simulink model "fourDiagonal"  (R2024a)
settings: Solver=VariableStepAuto  StartTime=0.0  StopTime=30.0  RelTol=1e-3
values from neighbouring files (symbols this model uses):
  b = fir1(filter_order, [low, high], 'band')    [load_params.m]
  lp_b = fir1(lp_filter_order, lowpass_high, 'low')    [load_params.m]
libraries: vrlib x1
settings Model: Creator=39351  LastModifiedBy=ozanpali
settings RTWCC: GPUComputeCapability=3.5

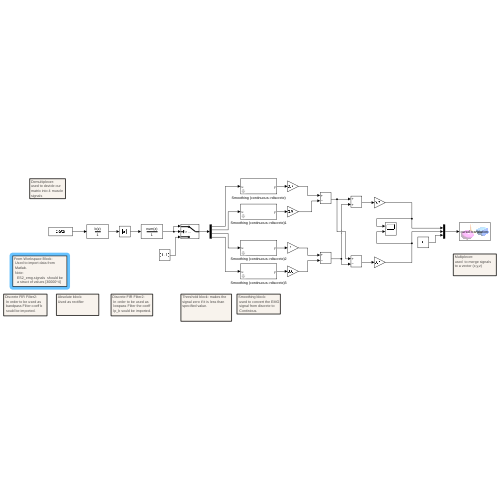
[thumbnail: Simulink's stored preview of the top-level diagram]
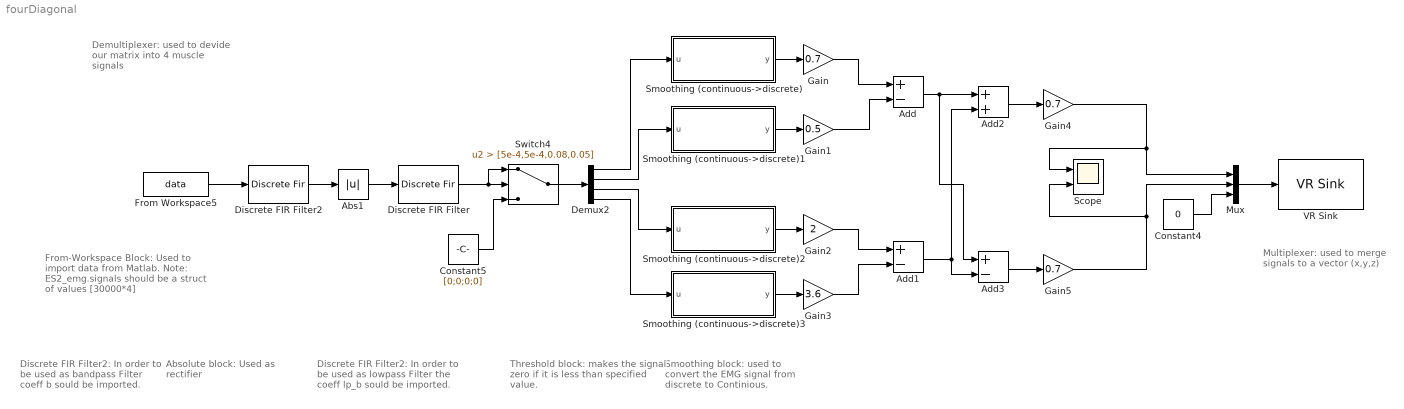
== system fourDiagonal ==
  note: Demultiplexer:
      | used to devide our
      | matrix into 4 muscle
      | signals
  note: Smoothing block:
      |  used to convert the EMG
      |  signal from discrete to
      |  Continious.
  note: Discrete FIR Filter2:
      |  In order to be used as
      |  lowpass Filter the coeff
      |  lp_b sould be imported.
  note: Absolute block:
      | Used as rectifier
  note: Discrete FIR Filter2:
      |  In order to be used as
      |  bandpass Filter coeff b
      |  sould be imported.
  note: Multiplexer:
      | used  to merge signals
      | to a vector (x,y,z)
  note: Threshold block: makes the
      | signal zero if it is less than
      | specified value.
  note: From-Workspace Block:
      |  Used to import data from
      |  Matlab.
      |  Note:
      |    ES2_emg.signals  should be
      |    a struct of values [30000*4]
  Abs1 : Abs  ZeroCross=off  OutDataTypeStr=double  SaturateOnIntegerOverflow=off
  Add : Sum  Inputs=+-
  Add1 : Sum  Inputs=+-
  Add2 : Sum
  Add3 : Sum  Inputs=+-
  Constant4 : Constant  Value=0
  Constant5 : Constant  Value=[0;0;0;0]
  Demux2 : Demux
  Discrete FIR Filter : DiscreteFir  Coefficients=lp_b  SampleTime=1/1000
  Discrete FIR Filter2 : DiscreteFir  Coefficients=b  SampleTime=1/1000
  From Workspace5 : FromWorkspace  VariableName=data  SampleTime=1/1000
  Gain : Gain  Gain=0.7
  Gain1 : Gain  Gain=0.5
  Gain2 : Gain  Gain=2
  Gain3 : Gain  Gain=3.6
  Gain4 : Gain  Gain=0.7
  Gain5 : Gain  Gain=0.7
  Mux : Mux  Inputs=3
  Scope : Scope  NumInputPorts=2
  Smoothing (continuous->discrete) : Subsystem  mask(Smoothing (continuous->discrete)){tsSmoothing=1, smoothing0=0}
      mask prompts: tsSmoothing "physmod:simscape:couplers:SimscapeNetworkCouplersLib:SmoothingTimeConstants_MP"; smoothing0 "physmod:simscape:couplers:SimscapeNetworkCouplersLib:InitialOutput_MP"
      mask help: physmod:simscape:couplers:SimscapeNetworkCouplersLib:Smoothingcontinuousdiscrete_MD
      mask Help: web([docroot '/physmod/simscape/ref/networkcouplersmoothingcontinuousdiscrete.html'])
      mask DialogControl tsSmoothing Prompt: Smoothing time constant (s)
      mask DialogControl smoothing0 Prompt: Initial output
  Smoothing (continuous->discrete)1 : Subsystem  mask(Smoothing (continuous->discrete)){tsSmoothing=1, smoothing0=0}
      mask prompts: tsSmoothing "physmod:simscape:couplers:SimscapeNetworkCouplersLib:SmoothingTimeConstants_MP"; smoothing0 "physmod:simscape:couplers:SimscapeNetworkCouplersLib:InitialOutput_MP"
      mask help: physmod:simscape:couplers:SimscapeNetworkCouplersLib:Smoothingcontinuousdiscrete_MD
      mask Help: web([docroot '/physmod/simscape/ref/networkcouplersmoothingcontinuousdiscrete.html'])
      mask DialogControl tsSmoothing Prompt: Smoothing time constant (s)
      mask DialogControl smoothing0 Prompt: Initial output
  Smoothing (continuous->discrete)2 : Subsystem  mask(Smoothing (continuous->discrete)){tsSmoothing=1.7, smoothing0=0}
      mask prompts: tsSmoothing "physmod:simscape:couplers:SimscapeNetworkCouplersLib:SmoothingTimeConstants_MP"; smoothing0 "physmod:simscape:couplers:SimscapeNetworkCouplersLib:InitialOutput_MP"
      mask help: physmod:simscape:couplers:SimscapeNetworkCouplersLib:Smoothingcontinuousdiscrete_MD
      mask Help: web([docroot '/physmod/simscape/ref/networkcouplersmoothingcontinuousdiscrete.html'])
      mask DialogControl tsSmoothing Prompt: Smoothing time constant (s)
      mask DialogControl smoothing0 Prompt: Initial output
  Smoothing (continuous->discrete)3 : Subsystem  mask(Smoothing (continuous->discrete)){tsSmoothing=1.2, smoothing0=0}
      mask prompts: tsSmoothing "physmod:simscape:couplers:SimscapeNetworkCouplersLib:SmoothingTimeConstants_MP"; smoothing0 "physmod:simscape:couplers:SimscapeNetworkCouplersLib:InitialOutput_MP"
      mask help: physmod:simscape:couplers:SimscapeNetworkCouplersLib:Smoothingcontinuousdiscrete_MD
      mask Help: web([docroot '/physmod/simscape/ref/networkcouplersmoothingcontinuousdiscrete.html'])
      mask DialogControl tsSmoothing Prompt: Smoothing time constant (s)
      mask DialogControl smoothing0 Prompt: Initial output
  Switch4 : Switch  Criteria=u2 > Threshold  Threshold=[5e-4,5e-4,0.08,0.05]  SaturateOnIntegerOverflow=off  InputSameDT=off
  VR Sink : vrlib/VR Sink  InstantiateOnLoad=on  SampleTime=0.1  ViewEnable=on  RemoteChange=off  RemoteView=off  FieldsWritten=cursor.translation.3.1.1.double  WorldFileName=8_palline_color.wrl  AutoView=off  VideoDimensions=[]  AllowVariableSize=off
  wires:
  Gain4/1 -> Mux/1, Scope/1
  Constant4/1 -> Mux/3
  Mux/1 -> VR Sink/1
  Smoothing (continuous->discrete)3/1(y) -> Gain3/1
  Smoothing (continuous->discrete)1/1(y) -> Gain1/1
  Smoothing (continuous->discrete)2/1(y) -> Gain2/1
  Gain1/1 -> Add/2
  Gain3/1 -> Add1/2
  Gain2/1 -> Add1/1
  Gain/1 -> Add/1
  Smoothing (continuous->discrete)/1(y) -> Gain/1
  Add/1 -> Add3/1, Add2/1
  Add1/1 -> Add2/2, Add3/2
  Add3/1 -> Gain5/1
  Add2/1 -> Gain4/1
  Gain5/1 -> Scope/2, Mux/2
  Discrete FIR Filter2/1 -> Abs1/1
  Abs1/1 -> Discrete FIR Filter/1
  From Workspace5/1 -> Discrete FIR Filter2/1
  Constant5/1 -> Switch4/3
  Switch4/1 -> Demux2/1
  Discrete FIR Filter/1 -> Switch4/2, Switch4/1
  Demux2/1 -> Smoothing (continuous->discrete)/1(u)
  Demux2/2 -> Smoothing (continuous->discrete)1/1(u)
  Demux2/3 -> Smoothing (continuous->discrete)2/1(u)
  Demux2/4 -> Smoothing (continuous->discrete)3/1(u)

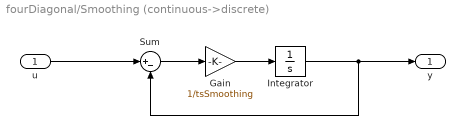
== system fourDiagonal/Smoothing (continuous->discrete) ==
  u : Inport
  Gain : Gain  Gain=1/tsSmoothing
  Integrator : Integrator  InitialCondition=smoothing0
  Sum : Sum  Inputs=|+-
  y : Outport
  wires:
  u/1 -> Sum/1
  Integrator/1 -> Sum/2, y/1
  Gain/1 -> Integrator/1
  Sum/1 -> Gain/1

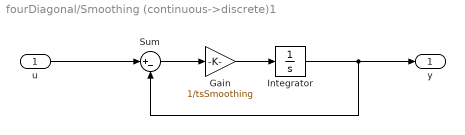
== system fourDiagonal/Smoothing (continuous->discrete)1 ==
  u : Inport
  Gain : Gain  Gain=1/tsSmoothing
  Integrator : Integrator  InitialCondition=smoothing0
  Sum : Sum  Inputs=|+-
  y : Outport
  wires:
  u/1 -> Sum/1
  Integrator/1 -> Sum/2, y/1
  Gain/1 -> Integrator/1
  Sum/1 -> Gain/1

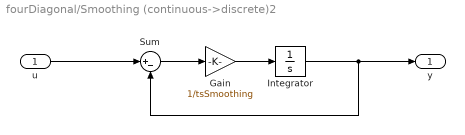
== system fourDiagonal/Smoothing (continuous->discrete)2 ==
  u : Inport
  Gain : Gain  Gain=1/tsSmoothing
  Integrator : Integrator  InitialCondition=smoothing0
  Sum : Sum  Inputs=|+-
  y : Outport
  wires:
  u/1 -> Sum/1
  Integrator/1 -> Sum/2, y/1
  Gain/1 -> Integrator/1
  Sum/1 -> Gain/1

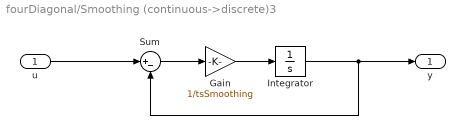
== system fourDiagonal/Smoothing (continuous->discrete)3 ==
  u : Inport
  Gain : Gain  Gain=1/tsSmoothing
  Integrator : Integrator  InitialCondition=smoothing0
  Sum : Sum  Inputs=|+-
  y : Outport
  wires:
  u/1 -> Sum/1
  Integrator/1 -> Sum/2, y/1
  Gain/1 -> Integrator/1
  Sum/1 -> Gain/1
